simulink model "sim1"  (R2020a)
settings: Solver=VariableStepAuto  StartTime=0.0  StopTime=0.01  RelTol=1e-3
values from neighbouring files (symbols this model uses):
  Kca = 0.10416    [be_trot.m]
  Kf = 1.45    [be_trot.m]
  Km = 1    [be_trot.m]
  T1 = 7.43e-5    (= 7.43e-05)    [be_trot.m]
  T2 = 4.84e-6    (= 4.84e-06)    [be_trot.m]
  Ti = K/(2*pi*400)    (= 0.0014422493619)    [be_trot.m]
  Tm = 0.002    [be_trot.m]
  Vbat = 12    [be_trot.m]
settings Model: Creator=lagrost  LastModifiedBy=lagrost

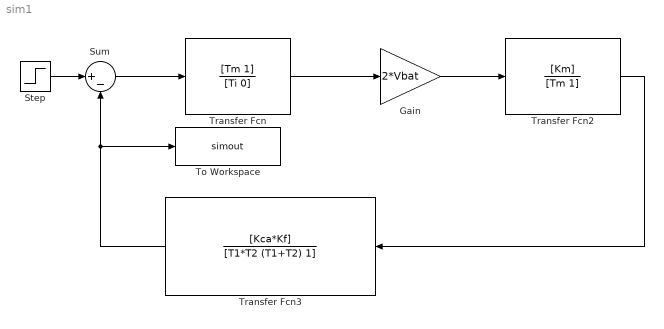
== system sim1 ==
  Gain : Gain  Gain=2*Vbat
  Step : Step  Time=0  After=1.65  SampleTime=0
  Sum : Sum  Inputs=|+-
  To Workspace : ToWorkspace  VariableName=simout  SaveFormat=Timeseries  SampleTime=-1
  Transfer Fcn : TransferFcn  Numerator=[Tm 1]  Denominator=[Ti 0]
  Transfer Fcn2 : TransferFcn  Numerator=[Km]  Denominator=[Tm 1]
  Transfer Fcn3 : TransferFcn  Numerator=[Kca*Kf]  Denominator=[T1*T2 (T1+T2) 1]
  wires:
  Transfer Fcn3/1 -> To Workspace/1, Sum/2
  Sum/1 -> Transfer Fcn/1
  Transfer Fcn/1 -> Gain/1
  Gain/1 -> Transfer Fcn2/1
  Transfer Fcn2/1 -> Transfer Fcn3/1
  Step/1 -> Sum/1
